simulink model "Implementacja_Smitha"  (R2022b)
settings: Solver=FixedStepAuto  StartTime=0.0  StopTime=40  RelTol=1e-3
values from neighbouring files (symbols this model uses):
  Ts = 0.15    [PID_OSWIETLENIE.m]    (also in PID_TEMPERATURA.m = 0.5)
undefined symbols (not defined in the file or in its folder): DiscIntNeverNeededParam, magnitude, Max_delay, MeanValue_random, Yr_step
libraries: slpidlib x1
settings Model: Creator=hpiet  LastModifiedBy=hpiet
settings SolverCC: AlgebraicLoopSolver=TrustRegion
settings DebuggingCC: UnconnectedInputMsg=warning  UnconnectedOutputMsg=warning  UnconnectedLineMsg=warning  SFMachineParentedDataDiag=warning
settings ModelReferenceCC: EnableRefExpFcnMdlSchedulingChecks=on
settings SFSimCC: CustomCodeUndefinedFunction=UseInterfaceOnly

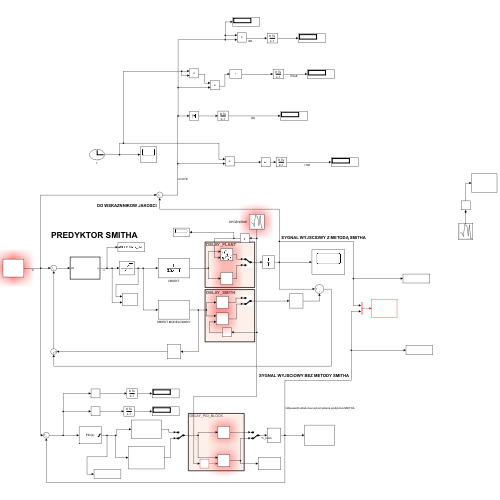
[thumbnail: Simulink's stored preview of the top-level diagram]
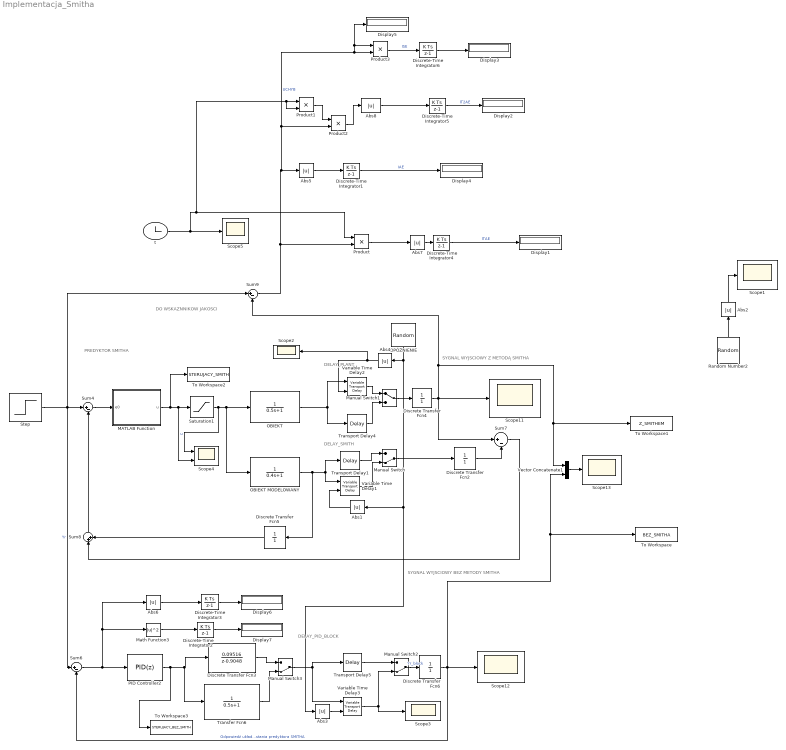
== system Implementacja_Smitha ==
  note: DO WSKAZNNIKOW JAKOSCI
  note: SYGNAL WYJSCIOWY Z METODĄ SMITHA
  note: SYGNAL WYJSCIOWY BEZ METODY SMITHA
  note: DELAY_PLANT
  note: DELAY_SMITH
  note: DELAY_PID_BLOCK
  note: PREDYKTOR SMITHA
  Abs{1..8} (8 alike) : Abs  SaturateOnIntegerOverflow=off
  Discrete Transfer Fcn{2,4..6} (4 alike) : DiscreteTransferFcn  Denominator=[1]  SampleTime=Ts
  Discrete Transfer Fcn3 : DiscreteTransferFcn  Numerator=[ 0.09516]  Denominator=[1 -0.9048]  SampleTime=Ts
  Discrete-Time Integrator{1..6} (6 alike) : DiscreteIntegrator  SampleTime=Ts  ICPrevOutput=DiscIntNeverNeededParam  ICPrevScaledInput=DiscIntNeverNeededParam
  Display{1..7} (7 alike) : Display
  MATLAB Function : MATLAB Function  TreatAsAtomicUnit=on
  Manual Switch : ManualSwitch  CurrentSetting=0
  Manual Switch1 : ManualSwitch
  Manual Switch2 : ManualSwitch  CurrentSetting=0
  Manual Switch3 : ManualSwitch  CurrentSetting=0
  Math Function3 : Math  Operator=magnitude^2  SignedPower=on
  OBIEKT : TransferFcn  Denominator=[0.5 1]
  OBIEKT MODELOWANY : TransferFcn  Denominator=[0.4 1]
  OPÓŻNIENIE : RandomNumber  Mean=MeanValue_random  Variance=0.0001  SampleTime=Ts
  PID Controller2 : slpidlib/PID Controller  Controller=PID  Form=Parallel  TimeDomain=Discrete-time  UseExternalTs=off  SampleTime=-1  IntegratorMethod=Backward Euler  FilterMethod=Backward Euler  ControllerParametersSource=internal  P=0.35265205372845  I=0.477399324378819  UseKiTs=off  D=0  N=0.588685123145228  UseFilter=on  TunerSelectOption=Transfer Function Based (PID Tuner App)  InitialConditionSource=internal  InitialConditionForIntegrator=0  InitialConditionForFilter=0  DifferentiatorICPrevScaledInput=0  ExternalReset=none  TrackingMode=off  Kt=1  LimitOutput=on  SatLimitsSource=internal  UpperSaturationLimit=inf  LowerSaturationLimit=-inf  LinearizeAsGain=off  AntiWindupMode=none  Kb=1  LimitIntegrator=off  UpperIntegratorSaturationLimit=inf  LowerIntegratorSaturationLimit=-inf  POutMin=[]  POutMax=[]  IOutMin=[]  IOutMax=[]  DOutMin=[]  DOutMax=[]  NOutMin=[]  NOutMax=[]  SumOutMin=[]  SumOutMax=[]  SaturationOutMin=[]  SaturationOutMax=[]  PParamMin=[]  PParamMax=[]  IParamMin=[]  IParamMax=[]  DParamMin=[]  DParamMax=[]  NParamMin=[]  NParamMax=[]  KbParamMin=[]  KbParamMax=[]  KtParamMin=[]  KtParamMax=[]  KbOutMin=[]  KbOutMax=[]  KtOutMin=[]  KtOutMax=[]  IntegratorOutMin=[]  IntegratorOutMax=[]  FilterOutMin=[]  FilterOutMax=[]  SumI1OutMin=[]  SumI1OutMax=[]  SumI2OutMin=[]  SumI2OutMax=[]  SumI3OutMin=[]  SumI3OutMax=[]  SumI4OutMin=[]  SumI4OutMax=[]  SumDOutMin=[]  SumDOutMax=[]  DifferentiatorOutMin=[]  DifferentiatorOutMax=[]  FilterDiffOutCoefMin=[]  FilterDiffOutCoefMax=[]  ReciprocalOutMin=[]  ReciprocalOutMax=[]  SumDenOutMin=[]  SumDenOutMax=[]  SumNumOutMin=[]  SumNumOutMax=[]  DivideOutMin=[]  DivideOutMax=[]  UdiffTsProdOutMin=[]  UdiffTsProdOutMax=[]  NTsProdOutMin=[]  NTsProdOutMax=[]  UintegralTsProdOutMin=[]  UintegralTsProdOutMax=[]  UngainTsProdOutMin=[]  UngainTsProdOutMax=[]  ClampingZeroOutDataTypeStr=Inherit: Inherit via back propagation  ClampingZeroOutMin=[]  ClampingZeroOutMax=[]  FilterDenConstantOutDataTypeStr=Inherit: Inherit via back propagation  FilterDenConstantOutMin=[]  FilterDenConstantOutMax=[]  PCopyOutDataTypeStr=Inherit: Inherit via back propagation  PCopyOutMin=[]  PCopyOutMax=[]  NCopyOutDataTypeStr=Inherit: Inherit via back propagation  NCopyOutMin=[]  NCopyOutMax=[]  IntegratorContinuousStateAttributes=''  IntegratorStateMustResolveToSignalObject=off  IntegratorRTWStateStorageClass=Auto  FilterContinuousStateAttributes=''  FilterStateMustResolveToSignalObject=off  FilterRTWStateStorageClass=Auto  ParallelPVariant=InternalParameters  IdealPVariant=Disabled  IVariant=InternalParameters  DVariant=InternalParameters  IntegratorVariant=Discrete  SatVariant=Enabled  AWVariant=Passthrough  PCopyVariant=Disabled  TRVariant=Disabled  FdbkBlocksVariant=Forward  IdealPFdbkVariant=Disabled  SatFdbkVariant=Disabled  DerivativeFilterVariant=BackwardEulerFilter  NVariant=InternalParameters  NCopyVariant=InternalParameters  FilterICVariant=InternalICsFilter  IntegratorICVariant=InternalICs  ExternalResetVariant=Disabled  TRSumVariant=Passthrough  SumFdbkVariant=Disabled  SumVariant=Sum_PID  TsampFilterVariant=InternalTs  TsampNgainVariant=Passthrough  TsampIntegralVariant=Passthrough  ExternalSaturationOutDataTypeStr=Inherit: Same as second input
  Product{,1..3} (4 alike) : Product
  Random Number2 : RandomNumber  Mean=0.08  Variance=0.0001  SampleTime=0.01
  Saturation1 : Saturate  UpperLimit=1000  LowerLimit=0
  Scope{1..3,5,11..13} (7 alike) : Scope
  Scope4 : Scope  NumInputPorts=2
  Step : Step  Time=0  After=Yr_step  SampleTime=Ts
  Sum{4,6..7,9} (4 alike) : Sum  Inputs=|+-
  Sum8 : Sum  Inputs=|++
  To Workspace : ToWorkspace  VariableName=BEZ_SMITHA  SaveFormat=Timeseries  SampleTime=-1
  To Workspace1 : ToWorkspace  VariableName=Z_SMITHEM  SaveFormat=Timeseries  SampleTime=-1
  To Workspace2 : ToWorkspace  VariableName=STERUJACY_SMITH  SaveFormat=Timeseries  SampleTime=-1
  To Workspace3 : ToWorkspace  VariableName=STERUJACY_BEZ_SMITH  SaveFormat=Timeseries  SampleTime=-1
  Transfer Fcn6 : TransferFcn  Denominator=[0.5 1]
  Transport Delay1 : TransportDelay  DelayTime=Max_delay
  Transport Delay4 : TransportDelay  DelayTime=Max_delay
  Transport Delay5 : TransportDelay  DelayTime=Max_delay
  Variable Time Delay1 : VariableTransportDelay  MaximumDelay=Max_delay
  Variable Time Delay2 : VariableTransportDelay  MaximumDelay=Max_delay
  Variable Time Delay3 : VariableTransportDelay  MaximumDelay=Max_delay
  Vector Concatenate1 : Concatenate
  t : Clock
  wires:
  Sum6/1 -> PID Controller2/1, Abs6/1, Math Function3/1
  Vector Concatenate1/1 -> Scope13/1
  Transport Delay4/1 -> Manual Switch1/2
  Discrete-Time Integrator2/1 -> Display7/1
  OBIEKT/1 -> Transport Delay4/1, Variable Time Delay2/1
  Discrete-Time Integrator3/1 -> Display6/1
  PID Controller2/1 -> To Workspace3/1, Transfer Fcn6/1, Discrete Transfer Fcn3/1
  Step/1 -> Sum4/1, Sum9/1, Sum6/1  "Yr"
  Math Function3/1 -> Discrete-Time Integrator2/1
  Discrete-Time Integrator1/1 -> Display4/1  "IAE"
  Sum8/1 -> Sum4/2
  Abs5/1 -> Discrete-Time Integrator1/1
  Abs6/1 -> Discrete-Time Integrator3/1
  Saturation1/1 -> Scope4/1, OBIEKT/1, OBIEKT MODELOWANY/1
  Abs1/1 -> Variable Time Delay1/2
  Random Number2/1 -> Abs2/1
  Abs2/1 -> Scope1/1
  Manual Switch/1 -> Discrete Transfer Fcn2/1
  Transport Delay1/1 -> Manual Switch/1
  Variable Time Delay1/1 -> Manual Switch/2
  MATLAB Function/1(u) -> To Workspace2/1, Scope4/2, Saturation1/1  "u"
  Abs4/1 -> Variable Time Delay2/2, Scope2/1
  Variable Time Delay2/1 -> Manual Switch1/1
  Manual Switch1/1 -> Discrete Transfer Fcn4/1
  Sum4/1 -> MATLAB Function/1(e0)
  Manual Switch3/1 -> Variable Time Delay3/1, Transport Delay5/1
  OPÓŻNIENIE/1 -> Abs3/1, Abs1/1, Abs4/1
  Abs3/1 -> Variable Time Delay3/2
  Transport Delay5/1 -> Manual Switch2/1
  Variable Time Delay3/1 -> Scope3/1, Manual Switch2/2
  Manual Switch2/1 -> Discrete Transfer Fcn6/1  "Yr_block"
  Sum7/1 -> Sum8/1
  OBIEKT MODELOWANY/1 -> Discrete Transfer Fcn5/1, Variable Time Delay1/1, Transport Delay1/1
  Discrete Transfer Fcn3/1 -> Manual Switch3/1
  Transfer Fcn6/1 -> Manual Switch3/2
  Discrete Transfer Fcn2/1 -> Sum7/2
  Discrete Transfer Fcn4/1 -> Sum7/1, Scope11/1, Vector Concatenate1/1, To Workspace1/1, Sum9/2
  Discrete Transfer Fcn5/1 -> Sum8/2
  Discrete Transfer Fcn6/1 -> Sum6/2, To Workspace/1, Vector Concatenate1/2, Scope12/1  "Odpowiedź układu bez wykorzystania predyktora SMITHA"
  t/1 -> Product1/2, Product1/1, Product/1, Scope5/1
  Abs8/1 -> Discrete-Time Integrator5/1
  Sum9/1 -> Product/2, Product2/2, Display5/1, Product3/1, Product3/2, Abs5/1  "UCHYB"
  Product/1 -> Abs7/1
  Abs7/1 -> Discrete-Time Integrator4/1
  Discrete-Time Integrator4/1 -> Display1/1  "ITAE"
  Discrete-Time Integrator5/1 -> Display2/1  "IT2AE"
  Product3/1 -> Discrete-Time Integrator6/1  "ISE"
  Discrete-Time Integrator6/1 -> Display3/1
  Product2/1 -> Abs8/1
  Product1/1 -> Product2/1

== matlab function Implementacja_Smitha/MATLAB Function ==
  settings: updateMethod=DISCRETE
  data: e0 input; u output
function u = PID(e0) 
persistent init e2 e1 u2 u1 ku1 ku2 ke0 ke1 ke2 ;
if isempty(init)
% Kp = 0.003577524793953;
% Ki =0.0263995998474549;
% Kd = -0.0003372324323117;
% FCoef = 3.2;
Ts=0.01; %czas próbki
Kp = 0.352652053728451;
Ki =0.477399324378819;
Kd = 0;
FCoef = 0.588685123145228;
e2=0;
e1=0;
u2=0;
u1=0;

a0 = (1 + FCoef * Ts);
a1 = -(2 + FCoef * Ts);
a2 = 1;

b0=Kp*(1+FCoef * Ts) + Ki*Ts*(1+ FCoef*Ts) + Kd*FCoef;
b1= -(Kp*(2+FCoef*Ts) + Ki*Ts + 2*Kd*FCoef);
b2=Kp + Kd * FCoef;

%uproszczenie równania
ku1=a1/a0;
ku2=a2/a0;
ke0=b0/a0;
ke1=b1/a0;
ke2=b2/a0;
init=1;
end

u0 = -(ku1*u1) - (ku2 * u2) + (ke0*e0) + (ke1*e1) + (ke2*e2);

e2=e1;
e1=e0;

%wyzerowanie u1 i u2 to część całkująca do zera
u2=u1;
u1=u0;

u=u0;
end
